simulink model "Buck_circuit_20discrete_identf"  (Simulink 8.8)
settings: Solver=ode8  StartTime=0.0  StopTime=0.5  FixedStep=0.000001  RelTol=1e-3  EnableMultiTasking=on
InitFcn:
  | Ts=4e-4;
libraries: powerlib x8, simulink x1
settings Model: Creator=KVRamana  LastModifiedBy=Chandan
settings OptimizationCC: ExpressionDepthLimit=2147483647
settings DebuggingCC: SolverPrmCheckMsg=warning

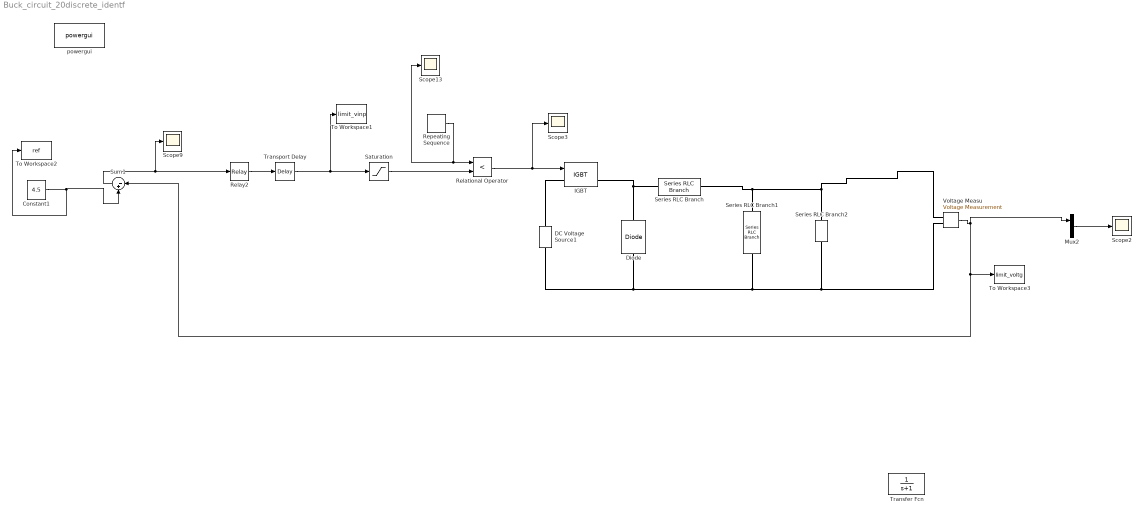
== system Buck_circuit_20discrete_identf ==
  Constant1 : Constant  Value=4.5
  DC Voltage Source1 : powerlib/Electrical Sources/DC Voltage Source  Amplitude=7.9  Measurements=None
  Diode : powerlib/Power Electronics/Diode  Ron=0.001  Lon=0  Vf=0.8  IC=0  UseSnubber=off  Rs=500  Cs=250e-9  Measurements=off
  IGBT : powerlib/Power Electronics/IGBT  Ron=0.001  Lon=0  Vf=1  Tf=1e-6  Tt=2e-6  IC=0  Rs=1e5  Cs=inf  Measurements=on
  Mux2 : Mux  Inputs=2
  Relational Operator : RelationalOperator  Operator=<  OutDataTypeStr=boolean  RndMeth=Nearest
  Relay2 : Relay  OnSwitchValue=0  OffSwitchValue=0  OnOutputValue=0.8  OffOutputValue=-0.8
  Repeating Sequence : simulink/Sources/Repeating Sequence  rep_seq_t=[0 1/20e3]  rep_seq_y=[0 1]
  Saturation : Saturate  UpperLimit=1  LowerLimit=0
  Scope{2..3,9,13} (4 alike) : Scope
  Series RLC Branch : powerlib/Elements/Series RLC Branch  LConnTagsString=__new0  RConnTagsString=__new0  BranchType=RL  Resistance=0.12  Inductance=0.00056  SetiL0=off  InitialCurrent=0  Capacitance=1e-6  Setx0=off  InitialVoltage=0  Measurements=None
  Series RLC Branch1 : powerlib/Elements/Series RLC Branch  LConnTagsString=__new0  RConnTagsString=__new0  BranchType=RC  Resistance=0.365  Inductance=1e-3  SetiL0=off  InitialCurrent=0  Capacitance=0.000098  Setx0=off  InitialVoltage=0  Measurements=None
  Series RLC Branch2 : powerlib/Elements/Series RLC Branch  LConnTagsString=__new0  RConnTagsString=__new0  BranchType=R  Resistance=10  Inductance=1e-3  SetiL0=off  InitialCurrent=0  Capacitance=0.000098  Setx0=off  InitialVoltage=0  Measurements=None
  Sum1 : Sum  Inputs=|-+
  To Workspace1 : ToWorkspace  VariableName=limit_vinp  SaveFormat=Structure With Time  SampleTime=-1
  To Workspace2 : ToWorkspace  VariableName=ref  SaveFormat=Structure With Time  SampleTime=-1
  To Workspace3 : ToWorkspace  VariableName=limit_voltg  SaveFormat=Structure With Time  SampleTime=-1
  Transfer Fcn : TransferFcn  Denominator=[1 1]
  Transport Delay : TransportDelay  DelayTime=0.00005
  Voltage Measu : powerlib/Measurements/Voltage Measurement  PhasorSimulation=off  OutputType=Complex  PSBequivalent=0
  powergui : powerlib/powergui  Priority=1  SimulationMode=Continuous  SolverType=Tustin  SampleTime=0.00001  frequency=60  SPID=off  DisableSnubberDevices=off  DisableRonSwitches=off  DisableVfSwitches=off  SwTol=0  DisplayEquations=off  Interpol=off  ExternalGateDelay=off  methode=off  Ts=0  FunctionMessages=off  echomessages=off  HookPort=off  EnableUseOfTLC=off  x0status=blocks  frequencyindice=0  Pbase=100e6  ErrMax=1e-4  Iterations=50  UnitsV=kV  UnitsW=MW  buscounter=0  RestoreLinks=warning  ResistiveCurrentMeasurement=off  Frange=[0:2:500]  Ylog=off  Xlog=on  ShowGrid=off  save=off  variable=ZData  structure=0  ZoomFFT=off  StartTime=0.0  cycles=1  DisplayStyle=1  fundamental=60  FreqAxis=off  MaxFrequency=1000  frequencyindicesteady=1  RmsSteady=1  display=off
  wires:
  Voltage Measu/1 -> Mux2/1, Sum1/1, To Workspace3/1
  Repeating Sequence/1 -> Relational Operator/1, Scope13/1
  Sum1/1 -> Scope9/1, Relay2/1
  Relational Operator/1 -> Scope3/1, IGBT/1
  Saturation/1 -> Relational Operator/2
  Constant1/1 -> Sum1/2, To Workspace2/1
  Mux2/1 -> Scope2/1
  Transport Delay/1 -> To Workspace1/1, Saturation/1
  Relay2/1 -> Transport Delay/1
  connections:
  IGBT/LConn1 -- DC Voltage Source1/RConn1
  Voltage Measu/LConn2 -- Diode/LConn1 -- DC Voltage Source1/LConn1 -- Series RLC Branch1/RConn1 -- Series RLC Branch2/RConn1
  Series RLC Branch/LConn1 -- IGBT/RConn1 -- Diode/RConn1
  Series RLC Branch1/LConn1 -- Voltage Measu/LConn1 -- Series RLC Branch2/LConn1 -- Series RLC Branch/RConn1
